simulink model "gm_uz_9ph_pmsm_model"  (R2021a)
settings: Solver=FixedStepAuto  StartTime=0.0  StopTime=.5  RelTol=1e-3
PreLoadFcn:
  | uz_pmsm_model_init_parameter
undefined symbols (not defined in the file or in its folder): friction_coefficient, inertia, k_i_d, k_p_d, k_p_q, L_d, L_o1, L_o2, L_q, L_x1, L_x2, L_y1, L_y2, L_zero, polepair, psi_pm, R_1, static_friction_torque
libraries: hdlmdlgenlib x220, hdlsllib x18, pid_lib x2, simulink x2
(part 2 of 3)

== system gm_uz_9ph_pmsm_model/uz_pmsm_model_9ph/Data Type Conversion11 ==
  In1 : Inport
  Data Type Conversion11 : DataTypeConversion  OutDataTypeStr=single  RndMeth=Nearest  SampleTime=1e-06
  Out1 : Outport
  wires:
  In1/1 -> Data Type Conversion11/1
  Data Type Conversion11/1 -> Out1/1

== system gm_uz_9ph_pmsm_model/uz_pmsm_model_9ph/Data Type Conversion111 ==
  In1 : Inport
  Data Type Conversion111 : DataTypeConversion  OutDataTypeStr=double  RndMeth=Nearest  SampleTime=1e-06
  Out1 : Outport
  wires:
  In1/1 -> Data Type Conversion111/1
  Data Type Conversion111/1 -> Out1/1

== system gm_uz_9ph_pmsm_model/uz_pmsm_model_9ph/Data Type Conversion12 ==
  In1 : Inport
  Data Type Conversion12 : DataTypeConversion  OutDataTypeStr=double  RndMeth=Nearest  SampleTime=1e-06
  Out1 : Outport
  wires:
  In1/1 -> Data Type Conversion12/1
  Data Type Conversion12/1 -> Out1/1

== system gm_uz_9ph_pmsm_model/uz_pmsm_model_9ph/Data Type Conversion121 ==
  In1 : Inport
  Data Type Conversion121 : DataTypeConversion  OutDataTypeStr=double  RndMeth=Nearest  SampleTime=1e-06
  Out1 : Outport
  wires:
  In1/1 -> Data Type Conversion121/1
  Data Type Conversion121/1 -> Out1/1

== system gm_uz_9ph_pmsm_model/uz_pmsm_model_9ph/Data Type Conversion15 ==
  In1 : Inport
  Data Type Conversion15 : DataTypeConversion  OutDataTypeStr=single  RndMeth=Nearest  SampleTime=1e-06
  Out1 : Outport
  wires:
  In1/1 -> Data Type Conversion15/1
  Data Type Conversion15/1 -> Out1/1

== system gm_uz_9ph_pmsm_model/uz_pmsm_model_9ph/Data Type Conversion16 ==
  In1 : Inport
  Data Type Conversion16 : DataTypeConversion  OutDataTypeStr=single  RndMeth=Nearest  SampleTime=1e-06
  Out1 : Outport
  wires:
  In1/1 -> Data Type Conversion16/1
  Data Type Conversion16/1 -> Out1/1

== system gm_uz_9ph_pmsm_model/uz_pmsm_model_9ph/Data Type Conversion17 ==
  In1 : Inport
  Data Type Conversion17 : DataTypeConversion  OutDataTypeStr=single  RndMeth=Nearest  SampleTime=1e-06
  Out1 : Outport
  wires:
  In1/1 -> Data Type Conversion17/1
  Data Type Conversion17/1 -> Out1/1

== system gm_uz_9ph_pmsm_model/uz_pmsm_model_9ph/Data Type Conversion18 ==
  In1 : Inport
  Data Type Conversion18 : DataTypeConversion  OutDataTypeStr=single  RndMeth=Nearest  SampleTime=1e-06
  Out1 : Outport
  wires:
  In1/1 -> Data Type Conversion18/1
  Data Type Conversion18/1 -> Out1/1

== system gm_uz_9ph_pmsm_model/uz_pmsm_model_9ph/Data Type Conversion19 ==
  In1 : Inport
  Data Type Conversion19 : DataTypeConversion  OutDataTypeStr=double  RndMeth=Nearest  SampleTime=1e-06
  Out1 : Outport
  wires:
  In1/1 -> Data Type Conversion19/1
  Data Type Conversion19/1 -> Out1/1

== system gm_uz_9ph_pmsm_model/uz_pmsm_model_9ph/Data Type Conversion2 ==
  In1 : Inport
  Data Type Conversion2 : DataTypeConversion  OutDataTypeStr=double  RndMeth=Nearest  SampleTime=1e-06
  Out1 : Outport
  wires:
  In1/1 -> Data Type Conversion2/1
  Data Type Conversion2/1 -> Out1/1

== system gm_uz_9ph_pmsm_model/uz_pmsm_model_9ph/Data Type Conversion21 ==
  In1 : Inport
  Data Type Conversion21 : DataTypeConversion  OutDataTypeStr=double  RndMeth=Nearest  SampleTime=1e-06
  Out1 : Outport
  wires:
  In1/1 -> Data Type Conversion21/1
  Data Type Conversion21/1 -> Out1/1

== system gm_uz_9ph_pmsm_model/uz_pmsm_model_9ph/Data Type Conversion26 ==
  In1 : Inport
  Data Type Conversion26 : DataTypeConversion  OutDataTypeStr=single  RndMeth=Nearest  SampleTime=1e-06
  Out1 : Outport
  wires:
  In1/1 -> Data Type Conversion26/1
  Data Type Conversion26/1 -> Out1/1

== system gm_uz_9ph_pmsm_model/uz_pmsm_model_9ph/Data Type Conversion3 ==
  In1 : Inport
  Data Type Conversion3 : DataTypeConversion  OutDataTypeStr=double  RndMeth=Nearest  SampleTime=1e-06
  Out1 : Outport
  wires:
  In1/1 -> Data Type Conversion3/1
  Data Type Conversion3/1 -> Out1/1

== system gm_uz_9ph_pmsm_model/uz_pmsm_model_9ph/Data Type Conversion30 ==
  In1 : Inport
  Data Type Conversion30 : DataTypeConversion  OutDataTypeStr=single  RndMeth=Nearest  SampleTime=1e-06
  Out1 : Outport
  wires:
  In1/1 -> Data Type Conversion30/1
  Data Type Conversion30/1 -> Out1/1

== system gm_uz_9ph_pmsm_model/uz_pmsm_model_9ph/Data Type Conversion31 ==
  In1 : Inport
  Data Type Conversion31 : DataTypeConversion  OutDataTypeStr=fixdt(1, 25, 12)  RndMeth=Nearest  SampleTime=1e-06
  Out1 : Outport
  wires:
  In1/1 -> Data Type Conversion31/1
  Data Type Conversion31/1 -> Out1/1

== system gm_uz_9ph_pmsm_model/uz_pmsm_model_9ph/Data Type Conversion32 ==
  In1 : Inport
  Data Type Conversion32 : DataTypeConversion  OutDataTypeStr=double  RndMeth=Nearest  SampleTime=1e-06
  Out1 : Outport
  wires:
  In1/1 -> Data Type Conversion32/1
  Data Type Conversion32/1 -> Out1/1

== system gm_uz_9ph_pmsm_model/uz_pmsm_model_9ph/Data Type Conversion4 ==
  In1 : Inport
  Data Type Conversion4 : DataTypeConversion  OutDataTypeStr=double  RndMeth=Nearest  SampleTime=1e-06
  Out1 : Outport
  wires:
  In1/1 -> Data Type Conversion4/1
  Data Type Conversion4/1 -> Out1/1

== system gm_uz_9ph_pmsm_model/uz_pmsm_model_9ph/Data Type Conversion41 ==
  In1 : Inport
  Data Type Conversion41 : DataTypeConversion  OutDataTypeStr=double  RndMeth=Nearest  SampleTime=1e-06
  Out1 : Outport
  wires:
  In1/1 -> Data Type Conversion41/1
  Data Type Conversion41/1 -> Out1/1

== system gm_uz_9ph_pmsm_model/uz_pmsm_model_9ph/Data Type Conversion5 ==
  In1 : Inport
  Data Type Conversion5 : DataTypeConversion  OutDataTypeStr=double  RndMeth=Nearest  SampleTime=1e-06
  Out1 : Outport
  wires:
  In1/1 -> Data Type Conversion5/1
  Data Type Conversion5/1 -> Out1/1

== system gm_uz_9ph_pmsm_model/uz_pmsm_model_9ph/Data Type Conversion51 ==
  In1 : Inport
  Data Type Conversion51 : DataTypeConversion  OutDataTypeStr=double  RndMeth=Nearest  SampleTime=1e-06
  Out1 : Outport
  wires:
  In1/1 -> Data Type Conversion51/1
  Data Type Conversion51/1 -> Out1/1

== system gm_uz_9ph_pmsm_model/uz_pmsm_model_9ph/Data Type Conversion6 ==
  In1 : Inport
  Data Type Conversion6 : DataTypeConversion  OutDataTypeStr=single  RndMeth=Nearest  SampleTime=1e-06
  Out1 : Outport
  wires:
  In1/1 -> Data Type Conversion6/1
  Data Type Conversion6/1 -> Out1/1

== system gm_uz_9ph_pmsm_model/uz_pmsm_model_9ph/Data Type Conversion61 ==
  In1 : Inport
  Data Type Conversion61 : DataTypeConversion  OutDataTypeStr=double  RndMeth=Nearest  SampleTime=1e-06
  Out1 : Outport
  wires:
  In1/1 -> Data Type Conversion61/1
  Data Type Conversion61/1 -> Out1/1

== system gm_uz_9ph_pmsm_model/uz_pmsm_model_9ph/Data Type Conversion71 ==
  In1 : Inport
  Data Type Conversion71 : DataTypeConversion  OutDataTypeStr=double  RndMeth=Nearest  SampleTime=1e-06
  Out1 : Outport
  wires:
  In1/1 -> Data Type Conversion71/1
  Data Type Conversion71/1 -> Out1/1

== system gm_uz_9ph_pmsm_model/uz_pmsm_model_9ph/Data Type Conversion8 ==
  In1 : Inport
  Data Type Conversion8 : DataTypeConversion  OutDataTypeStr=double  RndMeth=Nearest  SampleTime=1e-06
  Out1 : Outport
  wires:
  In1/1 -> Data Type Conversion8/1
  Data Type Conversion8/1 -> Out1/1

== system gm_uz_9ph_pmsm_model/uz_pmsm_model_9ph/Data Type Conversion9 ==
  In1 : Inport
  Data Type Conversion9 : DataTypeConversion  OutDataTypeStr=double  RndMeth=Nearest  SampleTime=1e-06
  Out1 : Outport
  wires:
  In1/1 -> Data Type Conversion9/1
  Data Type Conversion9/1 -> Out1/1

== system gm_uz_9ph_pmsm_model/uz_pmsm_model_9ph/Data Type Conversion91 ==
  In1 : Inport
  Data Type Conversion91 : DataTypeConversion  OutDataTypeStr=double  RndMeth=Nearest  SampleTime=1e-06
  Out1 : Outport
  wires:
  In1/1 -> Data Type Conversion91/1
  Data Type Conversion91/1 -> Out1/1

== system gm_uz_9ph_pmsm_model/uz_pmsm_model_9ph/Divide ==
  In1 : Inport
  In2 : Inport  Port=2
  Divide : Product  Inputs=**  OutDataTypeStr=double  SampleTime=1e-06
  Out1 : Outport
  wires:
  In1/1 -> Divide/1
  In2/1 -> Divide/2
  Divide/1 -> Out1/1

== system gm_uz_9ph_pmsm_model/uz_pmsm_model_9ph/Divide1 ==
  In1 : Inport
  In2 : Inport  Port=2
  Divide1 : Product  Inputs=**  OutDataTypeStr=double  SampleTime=1e-06
  Out1 : Outport
  wires:
  In1/1 -> Divide1/1
  In2/1 -> Divide1/2
  Divide1/1 -> Out1/1

== system gm_uz_9ph_pmsm_model/uz_pmsm_model_9ph/Divide10 ==
  In1 : Inport
  In2 : Inport  Port=2
  Divide10 : Product  Inputs=**  OutDataTypeStr=double  SampleTime=1e-06
  Out1 : Outport
  wires:
  In1/1 -> Divide10/1
  In2/1 -> Divide10/2
  Divide10/1 -> Out1/1

== system gm_uz_9ph_pmsm_model/uz_pmsm_model_9ph/Divide11 ==
  In1 : Inport
  In2 : Inport  Port=2
  Divide11 : Product  Inputs=*/  OutDataTypeStr=double  SampleTime=1e-06
  Out1 : Outport
  wires:
  In1/1 -> Divide11/1
  In2/1 -> Divide11/2
  Divide11/1 -> Out1/1

== system gm_uz_9ph_pmsm_model/uz_pmsm_model_9ph/Divide111 ==
  In1 : Inport
  In2 : Inport  Port=2
  Divide111 : Product  Inputs=*/  OutDataTypeStr=double  SampleTime=1e-06
  Out1 : Outport
  wires:
  In1/1 -> Divide111/1
  In2/1 -> Divide111/2
  Divide111/1 -> Out1/1

== system gm_uz_9ph_pmsm_model/uz_pmsm_model_9ph/Divide12 ==
  In1 : Inport
  In2 : Inport  Port=2
  Divide12 : Product  Inputs=**  OutDataTypeStr=double  SampleTime=1e-06
  Out1 : Outport
  wires:
  In1/1 -> Divide12/1
  In2/1 -> Divide12/2
  Divide12/1 -> Out1/1

== system gm_uz_9ph_pmsm_model/uz_pmsm_model_9ph/Divide13 ==
  In1 : Inport
  In2 : Inport  Port=2
  Divide13 : Product  Inputs=*/  OutDataTypeStr=double  SampleTime=1e-06
  Out1 : Outport
  wires:
  In1/1 -> Divide13/1
  In2/1 -> Divide13/2
  Divide13/1 -> Out1/1

== system gm_uz_9ph_pmsm_model/uz_pmsm_model_9ph/Divide2 ==
  In1 : Inport
  In2 : Inport  Port=2
  Divide2 : Product  Inputs=**  OutDataTypeStr=double  SampleTime=1e-06
  Out1 : Outport
  wires:
  In1/1 -> Divide2/1
  In2/1 -> Divide2/2
  Divide2/1 -> Out1/1

== system gm_uz_9ph_pmsm_model/uz_pmsm_model_9ph/Divide3 ==
  In1 : Inport
  In2 : Inport  Port=2
  Divide3 : Product  Inputs=*/  OutDataTypeStr=double  SampleTime=1e-06
  Out1 : Outport
  wires:
  In1/1 -> Divide3/1
  In2/1 -> Divide3/2
  Divide3/1 -> Out1/1

== system gm_uz_9ph_pmsm_model/uz_pmsm_model_9ph/Divide4 ==
  In1 : Inport
  In2 : Inport  Port=2
  Divide4 : Product  Inputs=**  OutDataTypeStr=double  SampleTime=1e-06
  Out1 : Outport
  wires:
  In1/1 -> Divide4/1
  In2/1 -> Divide4/2
  Divide4/1 -> Out1/1

== system gm_uz_9ph_pmsm_model/uz_pmsm_model_9ph/Divide5 ==
  In1 : Inport
  In2 : Inport  Port=2
  Divide5 : Product  Inputs=*/  OutDataTypeStr=double  SampleTime=1e-06
  Out1 : Outport
  wires:
  In1/1 -> Divide5/1
  In2/1 -> Divide5/2
  Divide5/1 -> Out1/1

== system gm_uz_9ph_pmsm_model/uz_pmsm_model_9ph/Divide6 ==
  In1 : Inport
  In2 : Inport  Port=2
  Divide6 : Product  Inputs=**  OutDataTypeStr=double  SampleTime=1e-06
  Out1 : Outport
  wires:
  In1/1 -> Divide6/1
  In2/1 -> Divide6/2
  Divide6/1 -> Out1/1

== system gm_uz_9ph_pmsm_model/uz_pmsm_model_9ph/Divide7 ==
  In1 : Inport
  In2 : Inport  Port=2
  Divide7 : Product  Inputs=*/  OutDataTypeStr=double  SampleTime=1e-06
  Out1 : Outport
  wires:
  In1/1 -> Divide7/1
  In2/1 -> Divide7/2
  Divide7/1 -> Out1/1

== system gm_uz_9ph_pmsm_model/uz_pmsm_model_9ph/Divide8 ==
  In1 : Inport
  In2 : Inport  Port=2
  Divide8 : Product  Inputs=**  OutDataTypeStr=double  SampleTime=1e-06
  Out1 : Outport
  wires:
  In1/1 -> Divide8/1
  In2/1 -> Divide8/2
  Divide8/1 -> Out1/1

== system gm_uz_9ph_pmsm_model/uz_pmsm_model_9ph/Divide9 ==
  In1 : Inport
  In2 : Inport  Port=2
  Divide9 : Product  Inputs=*/  OutDataTypeStr=double  SampleTime=1e-06
  Out1 : Outport
  wires:
  In1/1 -> Divide9/1
  In2/1 -> Divide9/2
  Divide9/1 -> Out1/1

== system gm_uz_9ph_pmsm_model/uz_pmsm_model_9ph/Factor ==
  In1 : Inport
  In2 : Inport  Port=2
  Factor : Product  Inputs=**  OutDataTypeStr=double  SampleTime=1e-06
  Out1 : Outport
  wires:
  In1/1 -> Factor/1
  In2/1 -> Factor/2
  Factor/1 -> Out1/1

== system gm_uz_9ph_pmsm_model/uz_pmsm_model_9ph/Gain ==
  In1 : Inport
  In2 : Inport  Port=2
  Gain : Product  Inputs=**  OutDataTypeStr=double  SampleTime=1e-06
  Out1 : Outport
  wires:
  In1/1 -> Gain/1
  In2/1 -> Gain/2
  Gain/1 -> Out1/1

== system gm_uz_9ph_pmsm_model/uz_pmsm_model_9ph/Gain1 ==
  In1 : Inport
  In2 : Inport  Port=2
  Gain1 : Product  Inputs=**  OutDataTypeStr=double  SampleTime=1e-06
  Out1 : Outport
  wires:
  In1/1 -> Gain1/1
  In2/1 -> Gain1/2
  Gain1/1 -> Out1/1

== system gm_uz_9ph_pmsm_model/uz_pmsm_model_9ph/Gain10 ==
  In1 : Inport
  In2 : Inport  Port=2
  Gain10 : Product  Inputs=**  OutDataTypeStr=double  SampleTime=1e-06
  Out1 : Outport
  wires:
  In1/1 -> Gain10/1
  In2/1 -> Gain10/2
  Gain10/1 -> Out1/1

== system gm_uz_9ph_pmsm_model/uz_pmsm_model_9ph/Gain2 ==
  In1 : Inport
  In2 : Inport  Port=2
  Gain2 : Product  Inputs=**  OutDataTypeStr=double  SampleTime=1e-06
  Out1 : Outport
  wires:
  In1/1 -> Gain2/1
  In2/1 -> Gain2/2
  Gain2/1 -> Out1/1

== system gm_uz_9ph_pmsm_model/uz_pmsm_model_9ph/Gain3 ==
  In1 : Inport
  In2 : Inport  Port=2
  Gain3 : Product  Inputs=**  OutDataTypeStr=double  SampleTime=1e-06
  Out1 : Outport
  wires:
  In1/1 -> Gain3/1
  In2/1 -> Gain3/2
  Gain3/1 -> Out1/1

== system gm_uz_9ph_pmsm_model/uz_pmsm_model_9ph/Gain4 ==
  In1 : Inport
  In2 : Inport  Port=2
  Gain4 : Product  Inputs=**  OutDataTypeStr=double  SampleTime=1e-06
  Out1 : Outport
  wires:
  In1/1 -> Gain4/1
  In2/1 -> Gain4/2
  Gain4/1 -> Out1/1

== system gm_uz_9ph_pmsm_model/uz_pmsm_model_9ph/Gain5 ==
  In1 : Inport
  In2 : Inport  Port=2
  Gain5 : Product  Inputs=**  OutDataTypeStr=double  SampleTime=1e-06
  Out1 : Outport
  wires:
  In1/1 -> Gain5/1
  In2/1 -> Gain5/2
  Gain5/1 -> Out1/1

== system gm_uz_9ph_pmsm_model/uz_pmsm_model_9ph/Gain6 ==
  In1 : Inport
  In2 : Inport  Port=2
  Gain6 : Product  Inputs=**  OutDataTypeStr=double  SampleTime=1e-06
  Out1 : Outport
  wires:
  In1/1 -> Gain6/1
  In2/1 -> Gain6/2
  Gain6/1 -> Out1/1

== system gm_uz_9ph_pmsm_model/uz_pmsm_model_9ph/Gain7 ==
  In1 : Inport
  In2 : Inport  Port=2
  Gain7 : Product  Inputs=**  OutDataTypeStr=double  SampleTime=1e-06
  Out1 : Outport
  wires:
  In1/1 -> Gain7/1
  In2/1 -> Gain7/2
  Gain7/1 -> Out1/1

== system gm_uz_9ph_pmsm_model/uz_pmsm_model_9ph/Gain8 ==
  In1 : Inport
  In2 : Inport  Port=2
  Gain8 : Product  Inputs=**  OutDataTypeStr=double  SampleTime=1e-06
  Out1 : Outport
  wires:
  In1/1 -> Gain8/1
  In2/1 -> Gain8/2
  Gain8/1 -> Out1/1

== system gm_uz_9ph_pmsm_model/uz_pmsm_model_9ph/Gain9 ==
  In1 : Inport
  In2 : Inport  Port=2
  Gain9 : Product  Inputs=**  OutDataTypeStr=double  SampleTime=1e-06
  Out1 : Outport
  wires:
  In1/1 -> Gain9/1
  In2/1 -> Gain9/2
  Gain9/1 -> Out1/1

== system gm_uz_9ph_pmsm_model/uz_pmsm_model_9ph/Product ==
  In1 : Inport
  In2 : Inport  Port=2
  Product : Product  Inputs=**  OutDataTypeStr=double  SampleTime=1e-06
  Out1 : Outport
  wires:
  In1/1 -> Product/1
  In2/1 -> Product/2
  Product/1 -> Out1/1

== system gm_uz_9ph_pmsm_model/uz_pmsm_model_9ph/Product1 ==
  In1 : Inport
  In2 : Inport  Port=2
  Product1 : Product  Inputs=**  OutDataTypeStr=double  SampleTime=1e-06
  Out1 : Outport
  wires:
  In1/1 -> Product1/1
  In2/1 -> Product1/2
  Product1/1 -> Out1/1

== system gm_uz_9ph_pmsm_model/uz_pmsm_model_9ph/Product10 ==
  In1 : Inport
  In2 : Inport  Port=2
  Product10 : Product  Inputs=**  OutDataTypeStr=double  SampleTime=1e-06
  Out1 : Outport
  wires:
  In1/1 -> Product10/1
  In2/1 -> Product10/2
  Product10/1 -> Out1/1

== system gm_uz_9ph_pmsm_model/uz_pmsm_model_9ph/Product11 ==
  In1 : Inport
  In2 : Inport  Port=2
  Product11 : Product  Inputs=**  OutDataTypeStr=double  SampleTime=1e-06
  Out1 : Outport
  wires:
  In1/1 -> Product11/1
  In2/1 -> Product11/2
  Product11/1 -> Out1/1

== system gm_uz_9ph_pmsm_model/uz_pmsm_model_9ph/Product12 ==
  In1 : Inport
  In2 : Inport  Port=2
  Product12 : Product  Inputs=**  OutDataTypeStr=double  SampleTime=1e-06
  Out1 : Outport
  wires:
  In1/1 -> Product12/1
  In2/1 -> Product12/2
  Product12/1 -> Out1/1

== system gm_uz_9ph_pmsm_model/uz_pmsm_model_9ph/Product2 ==
  In1 : Inport
  In2 : Inport  Port=2
  Product2 : Product  Inputs=**  OutDataTypeStr=double  SampleTime=1e-06
  Out1 : Outport
  wires:
  In1/1 -> Product2/1
  In2/1 -> Product2/2
  Product2/1 -> Out1/1

== system gm_uz_9ph_pmsm_model/uz_pmsm_model_9ph/Product3 ==
  In1 : Inport
  In2 : Inport  Port=2
  Product3 : Product  Inputs=**  OutDataTypeStr=double  SampleTime=1e-06
  Out1 : Outport
  wires:
  In1/1 -> Product3/1
  In2/1 -> Product3/2
  Product3/1 -> Out1/1

== system gm_uz_9ph_pmsm_model/uz_pmsm_model_9ph/Product4 ==
  In1 : Inport
  In2 : Inport  Port=2
  Product4 : Product  Inputs=**  OutDataTypeStr=double  SampleTime=1e-06
  Out1 : Outport
  wires:
  In1/1 -> Product4/1
  In2/1 -> Product4/2
  Product4/1 -> Out1/1

== system gm_uz_9ph_pmsm_model/uz_pmsm_model_9ph/Product5 ==
  In1 : Inport
  In2 : Inport  Port=2
  Product5 : Product  Inputs=**  OutDataTypeStr=double  SampleTime=1e-06
  Out1 : Outport
  wires:
  In1/1 -> Product5/1
  In2/1 -> Product5/2
  Product5/1 -> Out1/1

== system gm_uz_9ph_pmsm_model/uz_pmsm_model_9ph/Product6 ==
  In1 : Inport
  In2 : Inport  Port=2
  Product6 : Product  Inputs=**  OutDataTypeStr=double  SampleTime=1e-06
  Out1 : Outport
  wires:
  In1/1 -> Product6/1
  In2/1 -> Product6/2
  Product6/1 -> Out1/1

== system gm_uz_9ph_pmsm_model/uz_pmsm_model_9ph/Product7 ==
  In1 : Inport
  In2 : Inport  Port=2
  Product7 : Product  Inputs=**  OutDataTypeStr=double  SampleTime=1e-06
  Out1 : Outport
  wires:
  In1/1 -> Product7/1
  In2/1 -> Product7/2
  Product7/1 -> Out1/1

== system gm_uz_9ph_pmsm_model/uz_pmsm_model_9ph/Product8 ==
  In1 : Inport
  In2 : Inport  Port=2
  Product8 : Product  Inputs=**  OutDataTypeStr=double  SampleTime=1e-06
  Out1 : Outport
  wires:
  In1/1 -> Product8/1
  In2/1 -> Product8/2
  Product8/1 -> Out1/1

== system gm_uz_9ph_pmsm_model/uz_pmsm_model_9ph/Product9 ==
  In1 : Inport
  In2 : Inport  Port=2
  Product9 : Product  Inputs=**  OutDataTypeStr=double  SampleTime=1e-06
  Out1 : Outport
  wires:
  In1/1 -> Product9/1
  In2/1 -> Product9/2
  Product9/1 -> Out1/1

== system gm_uz_9ph_pmsm_model/uz_pmsm_model_9ph/Sign1 ==
  In1 : Inport
  Sign1 : Signum  SampleTime=1e-06
  Out1 : Outport
  wires:
  In1/1 -> Sign1/1
  Sign1/1 -> Out1/1

== system gm_uz_9ph_pmsm_model/uz_pmsm_model_9ph/Sum ==
  In1 : Inport
  In2 : Inport  Port=2
  Sum : Sum  Inputs=+-  OutDataTypeStr=double  SampleTime=1e-06
  Out1 : Outport
  wires:
  In1/1 -> Sum/1
  In2/1 -> Sum/2
  Sum/1 -> Out1/1

== system gm_uz_9ph_pmsm_model/uz_pmsm_model_9ph/Sum1 ==
  In1 : Inport
  In2 : Inport  Port=2
  Sum1 : Sum  Inputs=+-  OutDataTypeStr=double  SampleTime=1e-06
  Out1 : Outport
  wires:
  In1/1 -> Sum1/1
  In2/1 -> Sum1/2
  Sum1/1 -> Out1/1

== system gm_uz_9ph_pmsm_model/uz_pmsm_model_9ph/Sum1_stage2 ==
  In1 : Inport
  In2 : Inport  Port=2
  Sum1_stage2 : Sum  Inputs=+-  OutDataTypeStr=double  SampleTime=1e-06
  Out1 : Outport
  wires:
  In1/1 -> Sum1_stage2/1
  In2/1 -> Sum1_stage2/2
  Sum1_stage2/1 -> Out1/1

== system gm_uz_9ph_pmsm_model/uz_pmsm_model_9ph/Sum1_stage3 ==
  In1 : Inport
  In2 : Inport  Port=2
  Sum1_stage3 : Sum  Inputs=+-  OutDataTypeStr=double  SampleTime=1e-06
  Out1 : Outport
  wires:
  In1/1 -> Sum1_stage3/1
  In2/1 -> Sum1_stage3/2
  Sum1_stage3/1 -> Out1/1

== system gm_uz_9ph_pmsm_model/uz_pmsm_model_9ph/Sum2 ==
  In1 : Inport
  In2 : Inport  Port=2
  Sum2 : Sum  Inputs=+-  OutDataTypeStr=double  SampleTime=1e-06
  Out1 : Outport
  wires:
  In1/1 -> Sum2/1
  In2/1 -> Sum2/2
  Sum2/1 -> Out1/1

== system gm_uz_9ph_pmsm_model/uz_pmsm_model_9ph/Sum3 ==
  In1 : Inport
  In2 : Inport  Port=2
  Sum3 : Sum  OutDataTypeStr=double  SampleTime=1e-06
  Out1 : Outport
  wires:
  In1/1 -> Sum3/1
  In2/1 -> Sum3/2
  Sum3/1 -> Out1/1

== system gm_uz_9ph_pmsm_model/uz_pmsm_model_9ph/Sum31 ==
  In1 : Inport
  In2 : Inport  Port=2
  Sum31 : Sum  OutDataTypeStr=double  SampleTime=1e-06
  Out1 : Outport
  wires:
  In1/1 -> Sum31/1
  In2/1 -> Sum31/2
  Sum31/1 -> Out1/1

== system gm_uz_9ph_pmsm_model/uz_pmsm_model_9ph/Sum310 ==
  In1 : Inport
  In2 : Inport  Port=2
  Sum310 : Sum  OutDataTypeStr=double  SampleTime=1e-06
  Out1 : Outport
  wires:
  In1/1 -> Sum310/1
  In2/1 -> Sum310/2
  Sum310/1 -> Out1/1

== system gm_uz_9ph_pmsm_model/uz_pmsm_model_9ph/Sum311 ==
  In1 : Inport
  In2 : Inport  Port=2
  Sum311 : Sum  Inputs=+-  OutDataTypeStr=double  SampleTime=1e-06
  Out1 : Outport
  wires:
  In1/1 -> Sum311/1
  In2/1 -> Sum311/2
  Sum311/1 -> Out1/1

== system gm_uz_9ph_pmsm_model/uz_pmsm_model_9ph/Sum32 ==
  In1 : Inport
  In2 : Inport  Port=2
  Sum32 : Sum  OutDataTypeStr=double  SampleTime=1e-06
  Out1 : Outport
  wires:
  In1/1 -> Sum32/1
  In2/1 -> Sum32/2
  Sum32/1 -> Out1/1

== system gm_uz_9ph_pmsm_model/uz_pmsm_model_9ph/Sum33 ==
  In1 : Inport
  In2 : Inport  Port=2
  Sum33 : Sum  OutDataTypeStr=double  SampleTime=1e-06
  Out1 : Outport
  wires:
  In1/1 -> Sum33/1
  In2/1 -> Sum33/2
  Sum33/1 -> Out1/1

== system gm_uz_9ph_pmsm_model/uz_pmsm_model_9ph/Sum34 ==
  In1 : Inport
  In2 : Inport  Port=2
  Sum34 : Sum  OutDataTypeStr=double  SampleTime=1e-06
  Out1 : Outport
  wires:
  In1/1 -> Sum34/1
  In2/1 -> Sum34/2
  Sum34/1 -> Out1/1

== system gm_uz_9ph_pmsm_model/uz_pmsm_model_9ph/Sum35 ==
  In1 : Inport
  In2 : Inport  Port=2
  Sum35 : Sum  OutDataTypeStr=double  SampleTime=1e-06
  Out1 : Outport
  wires:
  In1/1 -> Sum35/1
  In2/1 -> Sum35/2
  Sum35/1 -> Out1/1

== system gm_uz_9ph_pmsm_model/uz_pmsm_model_9ph/Sum36 ==
  In1 : Inport
  In2 : Inport  Port=2
  Sum36 : Sum  OutDataTypeStr=double  SampleTime=1e-06
  Out1 : Outport
  wires:
  In1/1 -> Sum36/1
  In2/1 -> Sum36/2
  Sum36/1 -> Out1/1

== system gm_uz_9ph_pmsm_model/uz_pmsm_model_9ph/Sum37 ==
  In1 : Inport
  In2 : Inport  Port=2
  Sum37 : Sum  OutDataTypeStr=double  SampleTime=1e-06
  Out1 : Outport
  wires:
  In1/1 -> Sum37/1
  In2/1 -> Sum37/2
  Sum37/1 -> Out1/1

== system gm_uz_9ph_pmsm_model/uz_pmsm_model_9ph/Sum38 ==
  In1 : Inport
  In2 : Inport  Port=2
  Sum38 : Sum  OutDataTypeStr=double  SampleTime=1e-06
  Out1 : Outport
  wires:
  In1/1 -> Sum38/1
  In2/1 -> Sum38/2
  Sum38/1 -> Out1/1

== system gm_uz_9ph_pmsm_model/uz_pmsm_model_9ph/Sum39 ==
  In1 : Inport
  In2 : Inport  Port=2
  Sum39 : Sum  OutDataTypeStr=double  SampleTime=1e-06
  Out1 : Outport
  wires:
  In1/1 -> Sum39/1
  In2/1 -> Sum39/2
  Sum39/1 -> Out1/1

== system gm_uz_9ph_pmsm_model/uz_pmsm_model_9ph/Sum5 ==
  In1 : Inport
  In2 : Inport  Port=2
  Sum5 : Sum  OutDataTypeStr=double  SampleTime=1e-06
  Out1 : Outport
  wires:
  In1/1 -> Sum5/1
  In2/1 -> Sum5/2
  Sum5/1 -> Out1/1

== system gm_uz_9ph_pmsm_model/uz_pmsm_model_9ph/Sum_stage2 ==
  In1 : Inport
  In2 : Inport  Port=2
  Sum_stage2 : Sum  Inputs=+-  OutDataTypeStr=double  SampleTime=1e-06
  Out1 : Outport
  wires:
  In1/1 -> Sum_stage2/1
  In2/1 -> Sum_stage2/2
  Sum_stage2/1 -> Out1/1

== system gm_uz_9ph_pmsm_model/uz_pmsm_model_9ph/Sum_stage3 ==
  In1 : Inport
  In2 : Inport  Port=2
  Sum_stage3 : Sum  OutDataTypeStr=double  SampleTime=1e-06
  Out1 : Outport
  wires:
  In1/1 -> Sum_stage3/1
  In2/1 -> Sum_stage3/2
  Sum_stage3/1 -> Out1/1

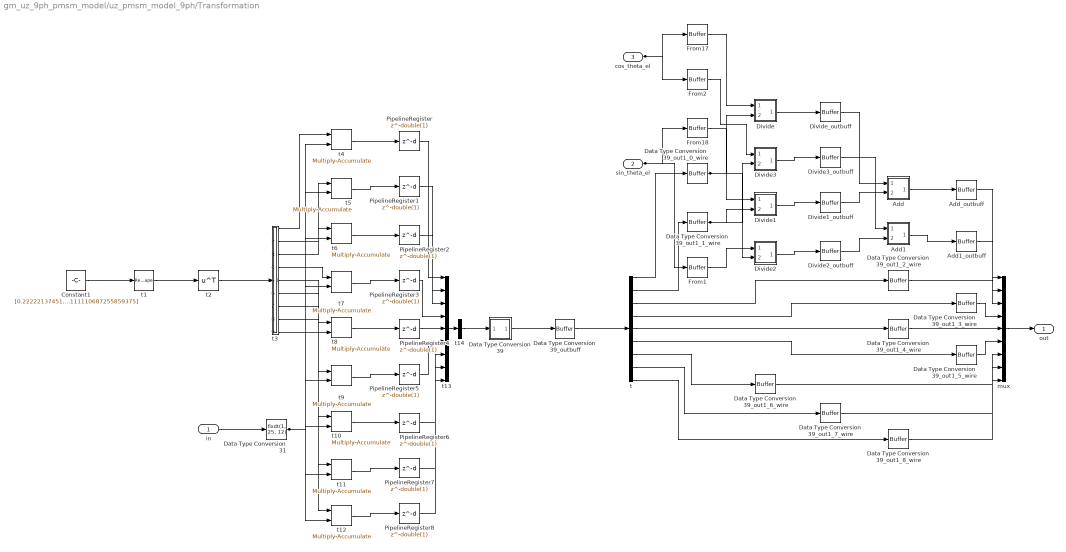
== system gm_uz_9ph_pmsm_model/uz_pmsm_model_9ph/Transformation ==
  in : Inport  OutDataTypeStr=fixdt(1, 25, 12)  PortDimensions=[9]  SampleTime=1e-06
  sin_theta_el : Inport  Port=2  OutDataTypeStr=single  SampleTime=1e-06
  cos_theta_el : Inport  Port=3  OutDataTypeStr=single  SampleTime=1e-06
  Add : Subsystem
      mask Display: disp('NFP\nadd');
  Add1 : Subsystem
      mask Display: disp('NFP\nadd');
  Add1_outbuff : hdlmdlgenlib/Buffer
      settings: SourceProductBaseCode=SL
  Add_outbuff : hdlmdlgenlib/Buffer
      settings: SourceProductBaseCode=SL
  Constant1 : Constant  Value=[0.22222137451171875;0;0.22222137451171875;0;0.22222137451171875;0;0.22222137451171875;0;0.111110687255859375;-0.111110687255859375;0.1924495697021484375;0.22222137451171875;0;-0.111110687255859375;-0.1924495697021484375;-0.111110687255859375;0.1924495697021484375;0.111110687255859375;-0.111110687255859375;-0.1924495697021484375;0.22222137451171875;0;-0.111110687255859375;0.1924495697021484375;-0.111110687255859375;-0.1924495697021484375;0.111110687255859375;0.208820343017578125;0.0760040283203125;0.111110687255859375;0.1924495697021484375;-0.0385875701904296875;0.218845367431640625;-0.1702327728271484375;0.142841339111328125;-0.111110687255859375;-0.1702327728271484375;0.142841339111328125;0.111110687255859375;0.1924495697021484375;0.208820343017578125;-0.0760040283203125;-0.0385875701904296875;-0.218845367431640625;-0.111110687255859375;-0.0385875701904296875;-0.218845367431640625;0.111110687255859375;0.1924495697021484375;-0.1702327728271484375;-0.142841339111328125;0.208820343017578125;0.0760040283203125;-0.111110687255859375;0.1702327728271484375;0.142841339111328125;-0.111110687255859375;0.1924495697021484375;-0.208820343017578125;-0.0760040283203125;0.0385875701904296875;-0.218845367431640625;0.111110687255859375;-0.208820343017578125;0.0760040283203125;-0.111110687255859375;0.1924495697021484375;0.0385875701904296875;0.218845367431640625;0.1702327728271484375;0.142841339111328125;0.111110687255859375;0.0385875701904296875;-0.218845367431640625;-0.111110687255859375;0.1924495697021484375;0.1702327728271484375;-0.142841339111328125;-0.208820343017578125;0.0760040283203125;0.111110687255859375]  OutDataTypeStr=fixdt(1, 18, 19)  SampleTime=1e-06
  Data Type Conversion31 : DataTypeConversion  OutDataTypeStr=fixdt(1, 25, 12)  RndMeth=Nearest  SampleTime=1e-06
  Data Type Conversion39 : Subsystem
      mask Display: disp('NFP\nconv');
  Data Type Conversion39_out1_0_wire : hdlmdlgenlib/Buffer
      settings: SourceProductBaseCode=SL
  Data Type Conversion39_out1_1_wire : hdlmdlgenlib/Buffer
      settings: SourceProductBaseCode=SL
  Data Type Conversion39_out1_2_wire : hdlmdlgenlib/Buffer
      settings: SourceProductBaseCode=SL
  Data Type Conversion39_out1_3_wire : hdlmdlgenlib/Buffer
      settings: SourceProductBaseCode=SL
  Data Type Conversion39_out1_4_wire : hdlmdlgenlib/Buffer
      settings: SourceProductBaseCode=SL
  Data Type Conversion39_out1_5_wire : hdlmdlgenlib/Buffer
      settings: SourceProductBaseCode=SL
  Data Type Conversion39_out1_6_wire : hdlmdlgenlib/Buffer
      settings: SourceProductBaseCode=SL
  Data Type Conversion39_out1_7_wire : hdlmdlgenlib/Buffer
      settings: SourceProductBaseCode=SL
  Data Type Conversion39_out1_8_wire : hdlmdlgenlib/Buffer
      settings: SourceProductBaseCode=SL
  Data Type Conversion39_outbuff : hdlmdlgenlib/Buffer
      settings: SourceProductBaseCode=SL
  Divide : Subsystem
      mask Display: disp('NFP\nmul');
  Divide1 : Subsystem
      mask Display: disp('NFP\nmul');
  Divide1_outbuff : hdlmdlgenlib/Buffer
      settings: SourceProductBaseCode=SL
  Divide2 : Subsystem
      mask Display: disp('NFP\nmul');
  Divide2_outbuff : hdlmdlgenlib/Buffer
      settings: SourceProductBaseCode=SL
  Divide3 : Subsystem
      mask Display: disp('NFP\nmul');
  Divide3_outbuff : hdlmdlgenlib/Buffer
      settings: SourceProductBaseCode=SL
  Divide_outbuff : hdlmdlgenlib/Buffer
      settings: SourceProductBaseCode=SL
  From{1..2,17..18} (4 alike) : hdlmdlgenlib/Buffer
      settings: SourceProductBaseCode=SL
  PipelineRegister{,1..8} (9 alike) : Delay  DelayLength=double(1)  InitialCondition=0  SampleTime=1e-06
  mux : Mux  Inputs=9
  t : Demux  Outputs=9
  t1 : Reshape  OutputDimensionality=Customize  OutputDimensions=[9,9]
  t{4..12} (9 alike) : hdlsllib/HDL Operations/Multiply-Accumulate  opMode=Vector  initValueSetting=Dialog  initValue=0  initValueSetting2=Dialog  initValue2=0  initValueSetting3=Dialog  initValue3=0  num_samples=2  RndMeth2=Floor  RndMeth3=Floor  OutDataTypeStr=fixdt(1, 43, 31)  datatype2=Inherit: Inherit via back propagation  datatype3=Inherit: Inherit via back propagation  validOut=on  endInandOut=on  startOut=on  countOut=on  dim=-1  DoSatur=off  parallel=off
      settings: SourceProductBaseCode=SL
  t13 : Mux  Inputs=9
  t14 : Concatenate  NumInputs=1  Mode=Multidimensional array  ConcatenateDimension=2
  t2 : Math  Operator=transpose  SaturateOnIntegerOverflow=on
  t3 : Subsystem
  out : Outport  SampleTime=1e-06
  wires:
  mux/1 -> out/1
  From1/1 -> Divide2/1(In1)
  From17/1 -> Divide/1(In1)
  Divide_outbuff/1 -> Add/1(In1)
  From18/1 -> Divide1/1(In1)
  Divide1_outbuff/1 -> Add/2(In2)
  From2/1 -> Divide3/1(In1)
  Divide3_outbuff/1 -> Add1/1(In1)
  t1/1 -> t2/1
  Data Type Conversion31/1 -> t12/2, t11/2, t10/2, t9/2, t8/2, t7/2, t6/2, t5/2, t4/2
  t14/1 -> Data Type Conversion39/1(In1)
  Data Type Conversion39_outbuff/1 -> t/1
  Data Type Conversion39_out1_0_wire/1 -> Divide2/2(In2), Divide/2(In2)
  Data Type Conversion39_out1_1_wire/1 -> Divide3/2(In2), Divide1/2(In2)
  Data Type Conversion39_out1_2_wire/1 -> mux/3
  Data Type Conversion39_out1_3_wire/1 -> mux/4
  Data Type Conversion39_out1_4_wire/1 -> mux/5
  Data Type Conversion39_out1_5_wire/1 -> mux/6
  Data Type Conversion39_out1_6_wire/1 -> mux/7
  Data Type Conversion39_out1_7_wire/1 -> mux/8
  Data Type Conversion39_out1_8_wire/1 -> mux/9
  Divide2_outbuff/1 -> Add1/2(In2)
  Add1_outbuff/1 -> mux/2
  Add_outbuff/1 -> mux/1
  t/1 -> Data Type Conversion39_out1_0_wire/1
  t/2 -> Data Type Conversion39_out1_1_wire/1
  t/3 -> Data Type Conversion39_out1_2_wire/1
  t/4 -> Data Type Conversion39_out1_3_wire/1
  t/5 -> Data Type Conversion39_out1_4_wire/1
  t/6 -> Data Type Conversion39_out1_5_wire/1
  t/7 -> Data Type Conversion39_out1_6_wire/1
  t/8 -> Data Type Conversion39_out1_7_wire/1
  t/9 -> Data Type Conversion39_out1_8_wire/1
  Constant1/1 -> t1/1
  t2/1 -> t3/1(in0)
  t3/1(out0) -> t4/1
  t3/2(out1) -> t5/1
  t3/3(out2) -> t6/1
  t3/4(out3) -> t7/1
  t3/5(out4) -> t8/1
  t3/6(out5) -> t9/1
  t3/7(out6) -> t10/1
  t3/8(out7) -> t11/1
  t3/9(out8) -> t12/1
  t13/1 -> t14/1
  PipelineRegister/1 -> t13/1
  PipelineRegister1/1 -> t13/2
  PipelineRegister2/1 -> t13/3
  PipelineRegister3/1 -> t13/4
  PipelineRegister4/1 -> t13/5
  PipelineRegister5/1 -> t13/6
  PipelineRegister6/1 -> t13/7
  PipelineRegister7/1 -> t13/8
  PipelineRegister8/1 -> t13/9
  Divide/1(Out1) -> Divide_outbuff/1
  Divide1/1(Out1) -> Divide1_outbuff/1
  Divide3/1(Out1) -> Divide3_outbuff/1
  Data Type Conversion39/1(Out1) -> Data Type Conversion39_outbuff/1
  Divide2/1(Out1) -> Divide2_outbuff/1
  Add1/1(Out1) -> Add1_outbuff/1
  Add/1(Out1) -> Add_outbuff/1
  in/1 -> Data Type Conversion31/1
  sin_theta_el/1 -> From1/1, From18/1
  cos_theta_el/1 -> From17/1, From2/1
  t4/1 -> PipelineRegister/1
  t5/1 -> PipelineRegister1/1
  t6/1 -> PipelineRegister2/1
  t7/1 -> PipelineRegister3/1
  t8/1 -> PipelineRegister4/1
  t9/1 -> PipelineRegister5/1
  t10/1 -> PipelineRegister6/1
  t11/1 -> PipelineRegister7/1
  t12/1 -> PipelineRegister8/1

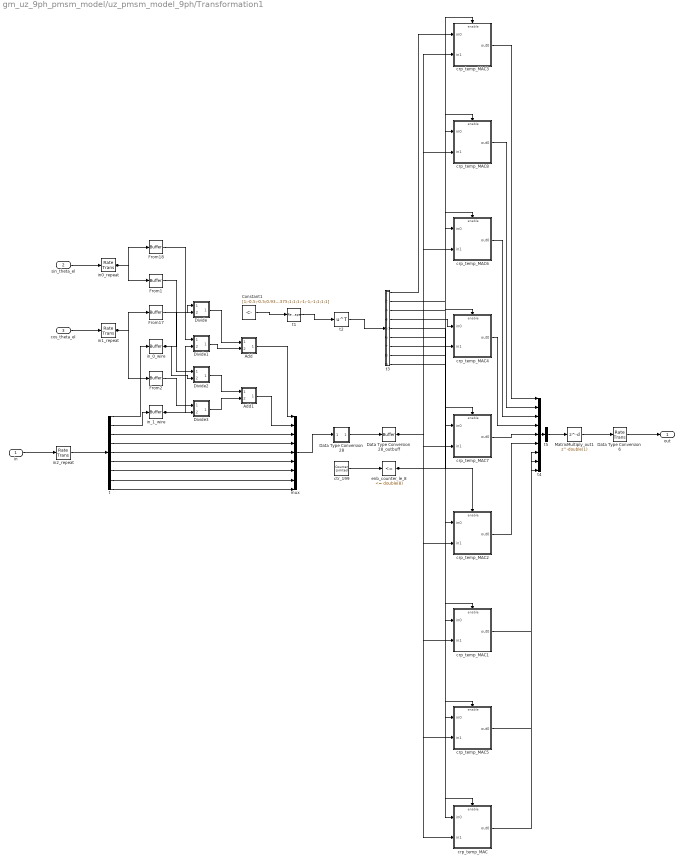
== system gm_uz_9ph_pmsm_model/uz_pmsm_model_9ph/Transformation1 ==
  in : Inport  OutDataTypeStr=single  PortDimensions=[9]  SampleTime=1e-06
  sin_theta_el : Inport  Port=2  OutDataTypeStr=single  SampleTime=1e-06
  cos_theta_el : Inport  Port=3  OutDataTypeStr=single  SampleTime=1e-06
  Add : Subsystem
      mask Display: disp('NFP\nadd');
  Add1 : Subsystem
      mask Display: disp('NFP\nadd');
  Constant1 : Constant  Value=[1;-0.5;-0.5;0.939697265625;-0.7660369873046875;-0.17364501953125;0.7660369873046875;-0.939697265625;0.17364501953125;0;0.86602783203125;-0.86602783203125;0.3420257568359375;0.642791748046875;-0.98480224609375;0.642791748046875;0.3420257568359375;-0.98480224609375;1;1;1;0.5;0.5;0.5;-0.5;-0.5;-0.5;0;0;0;0.86602783203125;0.86602783203125;0.86602783203125;0.86602783203125;0.86602783203125;0.86602783203125;1;-0.5;-0.5;-0.17364501953125;0.939697265625;-0.7660369873046875;-0.939697265625;0.17364501953125;0.7660369873046875;0;-0.86602783203125;0.86602783203125;0.98480224609375;-0.3420257568359375;-0.642791748046875;-0.3420257568359375;0.98480224609375;-0.642791748046875;1;-0.5;-0.5;-0.7660369873046875;-0.17364501953125;0.939697265625;0.17364501953125;0.7660369873046875;-0.939697265625;0;0.86602783203125;-0.86602783203125;0.642791748046875;-0.98480224609375;0.3420257568359375;-0.98480224609375;0.642791748046875;0.3420257568359375;1;1;1;-1;-1;-1;1;1;1]  OutDataTypeStr=fixdt(1, 18, 16)  SampleTime=5e-09
  Data Type Conversion28 : Subsystem
      mask Display: disp('NFP\nconv');
  Data Type Conversion28_outbuff : hdlmdlgenlib/Buffer
      settings: SourceProductBaseCode=SL
  Data Type Conversion6 : RateTransition  OutPortSampleTimeOpt=Multiple of input port sample time  OutPortSampleTimeMultiple=200
  Divide : Subsystem
      mask Display: disp('NFP\nmul');
  Divide1 : Subsystem
      mask Display: disp('NFP\nmul');
  Divide2 : Subsystem
      mask Display: disp('NFP\nmul');
  Divide3 : Subsystem
      mask Display: disp('NFP\nmul');
  From{1..2,17..18} (4 alike) : hdlmdlgenlib/Buffer
      settings: SourceProductBaseCode=SL
  MatrixMultiply_out1 : Delay  DelayLength=double(1)  InitialCondition=0  SampleTime=5e-09
  crp_temp_MAC : Subsystem
      settings: MinAlgLoopOccurrences=on
  crp_temp_MAC1 : Subsystem
      settings: MinAlgLoopOccurrences=on
  crp_temp_MAC2 : Subsystem
      settings: MinAlgLoopOccurrences=on
  crp_temp_MAC3 : Subsystem
      settings: MinAlgLoopOccurrences=on
  crp_temp_MAC4 : Subsystem
      settings: MinAlgLoopOccurrences=on
  crp_temp_MAC5 : Subsystem
      settings: MinAlgLoopOccurrences=on
  crp_temp_MAC6 : Subsystem
      settings: MinAlgLoopOccurrences=on
  crp_temp_MAC7 : Subsystem
      settings: MinAlgLoopOccurrences=on
  crp_temp_MAC8 : Subsystem
      settings: MinAlgLoopOccurrences=on
  ctr_199 : simulink/Sources/Counter Limited  uplimit=double(199)  tsamp=5e-09
  enb_counter_le_8 : simulink/Logic and Bit Operations/Compare To Constant  relop=<=  const=double(8)  OutDataTypeStr=boolean
  in0_repeat : RateTransition  Integrity=off  Deterministic=off  OutPortSampleTimeOpt=Multiple of input port sample time  OutPortSampleTimeMultiple=1/200
  in1_repeat : RateTransition  Integrity=off  Deterministic=off  OutPortSampleTimeOpt=Multiple of input port sample time  OutPortSampleTimeMultiple=1/200
  in2_repeat : RateTransition  Integrity=off  Deterministic=off  OutPortSampleTimeOpt=Multiple of input port sample time  OutPortSampleTimeMultiple=1/200
  in_0_wire : hdlmdlgenlib/Buffer
      settings: SourceProductBaseCode=SL
  in_1_wire : hdlmdlgenlib/Buffer
      settings: SourceProductBaseCode=SL
  mux : Mux  Inputs=9
  t : Demux  Outputs=9
  t1 : Reshape  OutputDimensionality=Customize  OutputDimensions=[9,9]
  t2 : Math  Operator=transpose  SaturateOnIntegerOverflow=on
  t3 : Subsystem
  t4 : Mux  Inputs=9
  t5 : Concatenate  NumInputs=1  Mode=Multidimensional array  ConcatenateDimension=2
  out : Outport  SampleTime=1e-06
  wires:
  in/1 -> in2_repeat/1
  sin_theta_el/1 -> in0_repeat/1
  cos_theta_el/1 -> in1_repeat/1
  Data Type Conversion6/1 -> out/1
  MatrixMultiply_out1/1 -> Data Type Conversion6/1
  in0_repeat/1 -> From1/1, From18/1
  in1_repeat/1 -> From17/1, From2/1
  in2_repeat/1 -> t/1
  t1/1 -> t2/1
  Data Type Conversion28_outbuff/1 -> crp_temp_MAC3/2(in1), crp_temp_MAC8/2(in1), crp_temp_MAC6/2(in1), crp_temp_MAC4/2(in1), crp_temp_MAC7/2(in1), crp_temp_MAC2/2(in1), crp_temp_MAC1/2(in1), crp_temp_MAC5/2(in1), crp_temp_MAC/2(in1)
  From1/1 -> Divide2/1(In1)
  From17/1 -> Divide/1(In1)
  From2/1 -> Divide3/1(In1)
  From18/1 -> Divide1/1(In1)
  in_0_wire/1 -> Divide2/2(In2), Divide/2(In2)
  in_1_wire/1 -> Divide1/2(In2), Divide3/2(In2)
  mux/1 -> Data Type Conversion28/1(In1)
  t5/1 -> MatrixMultiply_out1/1
  t/1 -> in_0_wire/1
  t/2 -> in_1_wire/1
  t/3 -> mux/3
  t/4 -> mux/4
  t/5 -> mux/5
  t/6 -> mux/6
  t/7 -> mux/7
  t/8 -> mux/8
  t/9 -> mux/9
  Constant1/1 -> t1/1
  t2/1 -> t3/1(in0)
  t3/1(out0) -> crp_temp_MAC3/1(in0)
  t3/2(out1) -> crp_temp_MAC8/1(in0)
  t3/3(out2) -> crp_temp_MAC6/1(in0)
  t3/4(out3) -> crp_temp_MAC4/1(in0)
  t3/5(out4) -> crp_temp_MAC7/1(in0)
  t3/6(out5) -> crp_temp_MAC2/1(in0)
  t3/7(out6) -> crp_temp_MAC1/1(in0)
  t3/8(out7) -> crp_temp_MAC5/1(in0)
  t3/9(out8) -> crp_temp_MAC/1(in0)
  crp_temp_MAC3/1(out0) -> t4/1
  crp_temp_MAC8/1(out0) -> t4/2
  crp_temp_MAC6/1(out0) -> t4/3
  crp_temp_MAC4/1(out0) -> t4/4
  crp_temp_MAC7/1(out0) -> t4/5
  crp_temp_MAC2/1(out0) -> t4/6
  crp_temp_MAC1/1(out0) -> t4/7
  crp_temp_MAC5/1(out0) -> t4/8
  crp_temp_MAC/1(out0) -> t4/9
  t4/1 -> t5/1
  Data Type Conversion28/1(Out1) -> Data Type Conversion28_outbuff/1
  Divide/1(Out1) -> Add/1(In1)
  Divide3/1(Out1) -> Add1/2(In2)
  Divide1/1(Out1) -> Add/2(In2)
  Divide2/1(Out1) -> Add1/1(In1)
  Add1/1(Out1) -> mux/2
  Add/1(Out1) -> mux/1
  enb_counter_le_8/1 -> crp_temp_MAC3/Enable, crp_temp_MAC8/Enable, crp_temp_MAC6/Enable, crp_temp_MAC4/Enable, crp_temp_MAC7/Enable, crp_temp_MAC2/Enable, crp_temp_MAC1/Enable, crp_temp_MAC5/Enable, crp_temp_MAC/Enable
  ctr_199/1 -> enb_counter_le_8/1

== system gm_uz_9ph_pmsm_model/uz_pmsm_model_9ph/Transformation/Add ==
  In1 : Inport
  In2 : Inport  Port=2
  Add : Sum  OutDataTypeStr=single  SampleTime=1e-06
  Out1 : Outport
  wires:
  In1/1 -> Add/1
  In2/1 -> Add/2
  Add/1 -> Out1/1

== system gm_uz_9ph_pmsm_model/uz_pmsm_model_9ph/Transformation/Add1 ==
  In1 : Inport
  In2 : Inport  Port=2
  Add1 : Sum  Inputs=+-  OutDataTypeStr=single  SampleTime=1e-06
  Out1 : Outport
  wires:
  In1/1 -> Add1/1
  In2/1 -> Add1/2
  Add1/1 -> Out1/1

== system gm_uz_9ph_pmsm_model/uz_pmsm_model_9ph/Transformation/Data Type Conversion39 ==
  In1 : Inport
  Data Type Conversion39 : DataTypeConversion  OutDataTypeStr=single  RndMeth=Nearest  SampleTime=1e-06
  Out1 : Outport
  wires:
  In1/1 -> Data Type Conversion39/1
  Data Type Conversion39/1 -> Out1/1

== system gm_uz_9ph_pmsm_model/uz_pmsm_model_9ph/Transformation/Divide ==
  In1 : Inport
  In2 : Inport  Port=2
  Divide : Product  Inputs=**  OutDataTypeStr=single  SampleTime=1e-06
  Out1 : Outport
  wires:
  In1/1 -> Divide/1
  In2/1 -> Divide/2
  Divide/1 -> Out1/1

== system gm_uz_9ph_pmsm_model/uz_pmsm_model_9ph/Transformation/Divide1 ==
  In1 : Inport
  In2 : Inport  Port=2
  Divide1 : Product  Inputs=**  OutDataTypeStr=single  SampleTime=1e-06
  Out1 : Outport
  wires:
  In1/1 -> Divide1/1
  In2/1 -> Divide1/2
  Divide1/1 -> Out1/1

== system gm_uz_9ph_pmsm_model/uz_pmsm_model_9ph/Transformation/Divide2 ==
  In1 : Inport
  In2 : Inport  Port=2
  Divide2 : Product  Inputs=**  OutDataTypeStr=single  SampleTime=1e-06
  Out1 : Outport
  wires:
  In1/1 -> Divide2/1
  In2/1 -> Divide2/2
  Divide2/1 -> Out1/1

== system gm_uz_9ph_pmsm_model/uz_pmsm_model_9ph/Transformation/Divide3 ==
  In1 : Inport
  In2 : Inport  Port=2
  Divide3 : Product  Inputs=**  OutDataTypeStr=single  SampleTime=1e-06
  Out1 : Outport
  wires:
  In1/1 -> Divide3/1
  In2/1 -> Divide3/2
  Divide3/1 -> Out1/1

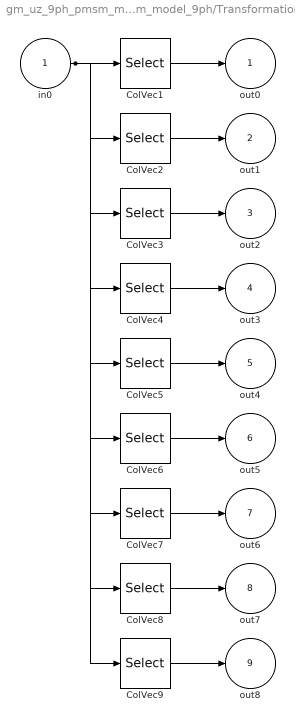
== system gm_uz_9ph_pmsm_model/uz_pmsm_model_9ph/Transformation/t3 ==
  in0 : Inport
  ColVec1 : Selector  NumberOfDimensions=2  IndexOptions=Select all,Index vector (dialog)  Indices=1,1  OutputSizes=1,1
  ColVec2 : Selector  NumberOfDimensions=2  IndexOptions=Select all,Index vector (dialog)  Indices=1,2  OutputSizes=1,1
  ColVec3 : Selector  NumberOfDimensions=2  IndexOptions=Select all,Index vector (dialog)  Indices=1,3  OutputSizes=1,1
  ColVec4 : Selector  NumberOfDimensions=2  IndexOptions=Select all,Index vector (dialog)  Indices=1,4  OutputSizes=1,1
  ColVec5 : Selector  NumberOfDimensions=2  IndexOptions=Select all,Index vector (dialog)  Indices=1,5  OutputSizes=1,1
  ColVec6 : Selector  NumberOfDimensions=2  IndexOptions=Select all,Index vector (dialog)  Indices=1,6  OutputSizes=1,1
  ColVec7 : Selector  NumberOfDimensions=2  IndexOptions=Select all,Index vector (dialog)  Indices=1,7  OutputSizes=1,1
  ColVec8 : Selector  NumberOfDimensions=2  IndexOptions=Select all,Index vector (dialog)  Indices=1,8  OutputSizes=1,1
  ColVec9 : Selector  NumberOfDimensions=2  IndexOptions=Select all,Index vector (dialog)  Indices=1,9  OutputSizes=1,1
  out0 : Outport
  out1 : Outport  Port=2
  out2 : Outport  Port=3
  out3 : Outport  Port=4
  out4 : Outport  Port=5
  out5 : Outport  Port=6
  out6 : Outport  Port=7
  out7 : Outport  Port=8
  out8 : Outport  Port=9
  wires:
  in0/1 -> ColVec1/1, ColVec2/1, ColVec3/1, ColVec4/1, ColVec5/1, ColVec6/1, ColVec7/1, ColVec8/1, ColVec9/1
  ColVec1/1 -> out0/1
  ColVec2/1 -> out1/1
  ColVec3/1 -> out2/1
  ColVec4/1 -> out3/1
  ColVec5/1 -> out4/1
  ColVec6/1 -> out5/1
  ColVec7/1 -> out6/1
  ColVec8/1 -> out7/1
  ColVec9/1 -> out8/1

== system gm_uz_9ph_pmsm_model/uz_pmsm_model_9ph/Transformation1/Add ==
  In1 : Inport
  In2 : Inport  Port=2
  Add : Sum  Inputs=+-  OutDataTypeStr=single  SampleTime=5e-09
  Out1 : Outport
  wires:
  In1/1 -> Add/1
  In2/1 -> Add/2
  Add/1 -> Out1/1

== system gm_uz_9ph_pmsm_model/uz_pmsm_model_9ph/Transformation1/Add1 ==
  In1 : Inport
  In2 : Inport  Port=2
  Add1 : Sum  OutDataTypeStr=single  SampleTime=5e-09
  Out1 : Outport
  wires:
  In1/1 -> Add1/1
  In2/1 -> Add1/2
  Add1/1 -> Out1/1

== system gm_uz_9ph_pmsm_model/uz_pmsm_model_9ph/Transformation1/Data Type Conversion28 ==
  In1 : Inport
  Data Type Conversion28 : DataTypeConversion  OutDataTypeStr=fixdt(1, 25, 12)  RndMeth=Nearest  SampleTime=5e-09
  Out1 : Outport
  wires:
  In1/1 -> Data Type Conversion28/1
  Data Type Conversion28/1 -> Out1/1

== system gm_uz_9ph_pmsm_model/uz_pmsm_model_9ph/Transformation1/Divide ==
  In1 : Inport
  In2 : Inport  Port=2
  Divide : Product  Inputs=**  OutDataTypeStr=single  SampleTime=5e-09
  Out1 : Outport
  wires:
  In1/1 -> Divide/1
  In2/1 -> Divide/2
  Divide/1 -> Out1/1

== system gm_uz_9ph_pmsm_model/uz_pmsm_model_9ph/Transformation1/Divide1 ==
  In1 : Inport
  In2 : Inport  Port=2
  Divide1 : Product  Inputs=**  OutDataTypeStr=single  SampleTime=5e-09
  Out1 : Outport
  wires:
  In1/1 -> Divide1/1
  In2/1 -> Divide1/2
  Divide1/1 -> Out1/1

== system gm_uz_9ph_pmsm_model/uz_pmsm_model_9ph/Transformation1/Divide2 ==
  In1 : Inport
  In2 : Inport  Port=2
  Divide2 : Product  Inputs=**  OutDataTypeStr=single  SampleTime=5e-09
  Out1 : Outport
  wires:
  In1/1 -> Divide2/1
  In2/1 -> Divide2/2
  Divide2/1 -> Out1/1

== system gm_uz_9ph_pmsm_model/uz_pmsm_model_9ph/Transformation1/Divide3 ==
  In1 : Inport
  In2 : Inport  Port=2
  Divide3 : Product  Inputs=**  OutDataTypeStr=single  SampleTime=5e-09
  Out1 : Outport
  wires:
  In1/1 -> Divide3/1
  In2/1 -> Divide3/2
  Divide3/1 -> Out1/1

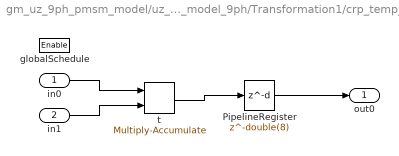
== system gm_uz_9ph_pmsm_model/uz_pmsm_model_9ph/Transformation1/crp_temp_MAC ==
  in0 : Inport  OutDataTypeStr=fixdt(1, 18, 16)  PortDimensions=[9 1]  SampleTime=5e-09
  in1 : Inport  Port=2  OutDataTypeStr=fixdt(1, 25, 12)  PortDimensions=[9]  SampleTime=5e-09
  globalSchedule : EnablePort  OutDataTypeStr=boolean
  PipelineRegister : Delay  DelayLength=double(8)  InitialCondition=0
  t : hdlsllib/HDL Operations/Multiply-Accumulate  opMode=Vector  initValueSetting=Dialog  initValue=0  initValueSetting2=Dialog  initValue2=0  initValueSetting3=Dialog  initValue3=0  num_samples=2  RndMeth2=Floor  RndMeth3=Floor  OutDataTypeStr=fixdt(1, 43, 28)  datatype2=Inherit: Inherit via back propagation  datatype3=Inherit: Inherit via back propagation  validOut=on  endInandOut=on  startOut=on  countOut=on  dim=-1  DoSatur=off  parallel=off
      settings: SourceProductBaseCode=SL
  out0 : Outport  OutDataTypeStr=fixdt(1, 43, 28)  SampleTime=5e-09  InitialOutput=0
  wires:
  PipelineRegister/1 -> out0/1
  in0/1 -> t/1
  in1/1 -> t/2
  t/1 -> PipelineRegister/1

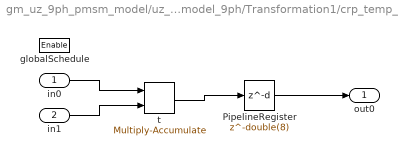
== system gm_uz_9ph_pmsm_model/uz_pmsm_model_9ph/Transformation1/crp_temp_MAC1 ==
  in0 : Inport  OutDataTypeStr=fixdt(1, 18, 16)  PortDimensions=[9 1]  SampleTime=5e-09
  in1 : Inport  Port=2  OutDataTypeStr=fixdt(1, 25, 12)  PortDimensions=[9]  SampleTime=5e-09
  globalSchedule : EnablePort  OutDataTypeStr=boolean
  PipelineRegister : Delay  DelayLength=double(8)  InitialCondition=0
  t : hdlsllib/HDL Operations/Multiply-Accumulate  opMode=Vector  initValueSetting=Dialog  initValue=0  initValueSetting2=Dialog  initValue2=0  initValueSetting3=Dialog  initValue3=0  num_samples=2  RndMeth2=Floor  RndMeth3=Floor  OutDataTypeStr=fixdt(1, 43, 28)  datatype2=Inherit: Inherit via back propagation  datatype3=Inherit: Inherit via back propagation  validOut=on  endInandOut=on  startOut=on  countOut=on  dim=-1  DoSatur=off  parallel=off
      settings: SourceProductBaseCode=SL
  out0 : Outport  OutDataTypeStr=fixdt(1, 43, 28)  SampleTime=5e-09  InitialOutput=0
  wires:
  PipelineRegister/1 -> out0/1
  in0/1 -> t/1
  in1/1 -> t/2
  t/1 -> PipelineRegister/1

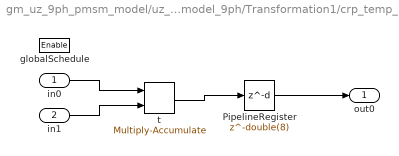
== system gm_uz_9ph_pmsm_model/uz_pmsm_model_9ph/Transformation1/crp_temp_MAC2 ==
  in0 : Inport  OutDataTypeStr=fixdt(1, 18, 16)  PortDimensions=[9 1]  SampleTime=5e-09
  in1 : Inport  Port=2  OutDataTypeStr=fixdt(1, 25, 12)  PortDimensions=[9]  SampleTime=5e-09
  globalSchedule : EnablePort  OutDataTypeStr=boolean
  PipelineRegister : Delay  DelayLength=double(8)  InitialCondition=0
  t : hdlsllib/HDL Operations/Multiply-Accumulate  opMode=Vector  initValueSetting=Dialog  initValue=0  initValueSetting2=Dialog  initValue2=0  initValueSetting3=Dialog  initValue3=0  num_samples=2  RndMeth2=Floor  RndMeth3=Floor  OutDataTypeStr=fixdt(1, 43, 28)  datatype2=Inherit: Inherit via back propagation  datatype3=Inherit: Inherit via back propagation  validOut=on  endInandOut=on  startOut=on  countOut=on  dim=-1  DoSatur=off  parallel=off
      settings: SourceProductBaseCode=SL
  out0 : Outport  OutDataTypeStr=fixdt(1, 43, 28)  SampleTime=5e-09  InitialOutput=0
  wires:
  PipelineRegister/1 -> out0/1
  in0/1 -> t/1
  in1/1 -> t/2
  t/1 -> PipelineRegister/1

== system gm_uz_9ph_pmsm_model/uz_pmsm_model_9ph/Transformation1/crp_temp_MAC3 ==
  in0 : Inport  OutDataTypeStr=fixdt(1, 18, 16)  PortDimensions=[9 1]  SampleTime=5e-09
  in1 : Inport  Port=2  OutDataTypeStr=fixdt(1, 25, 12)  PortDimensions=[9]  SampleTime=5e-09
  globalSchedule : EnablePort  OutDataTypeStr=boolean
  PipelineRegister : Delay  DelayLength=double(8)  InitialCondition=0
  t : hdlsllib/HDL Operations/Multiply-Accumulate  opMode=Vector  initValueSetting=Dialog  initValue=0  initValueSetting2=Dialog  initValue2=0  initValueSetting3=Dialog  initValue3=0  num_samples=2  RndMeth2=Floor  RndMeth3=Floor  OutDataTypeStr=fixdt(1, 43, 28)  datatype2=Inherit: Inherit via back propagation  datatype3=Inherit: Inherit via back propagation  validOut=on  endInandOut=on  startOut=on  countOut=on  dim=-1  DoSatur=off  parallel=off
      settings: SourceProductBaseCode=SL
  out0 : Outport  OutDataTypeStr=fixdt(1, 43, 28)  SampleTime=5e-09  InitialOutput=0
  wires:
  PipelineRegister/1 -> out0/1
  in0/1 -> t/1
  in1/1 -> t/2
  t/1 -> PipelineRegister/1

== system gm_uz_9ph_pmsm_model/uz_pmsm_model_9ph/Transformation1/crp_temp_MAC4 ==
  in0 : Inport  OutDataTypeStr=fixdt(1, 18, 16)  PortDimensions=[9 1]  SampleTime=5e-09
  in1 : Inport  Port=2  OutDataTypeStr=fixdt(1, 25, 12)  PortDimensions=[9]  SampleTime=5e-09
  globalSchedule : EnablePort  OutDataTypeStr=boolean
  PipelineRegister : Delay  DelayLength=double(8)  InitialCondition=0
  t : hdlsllib/HDL Operations/Multiply-Accumulate  opMode=Vector  initValueSetting=Dialog  initValue=0  initValueSetting2=Dialog  initValue2=0  initValueSetting3=Dialog  initValue3=0  num_samples=2  RndMeth2=Floor  RndMeth3=Floor  OutDataTypeStr=fixdt(1, 43, 28)  datatype2=Inherit: Inherit via back propagation  datatype3=Inherit: Inherit via back propagation  validOut=on  endInandOut=on  startOut=on  countOut=on  dim=-1  DoSatur=off  parallel=off
      settings: SourceProductBaseCode=SL
  out0 : Outport  OutDataTypeStr=fixdt(1, 43, 28)  SampleTime=5e-09  InitialOutput=0
  wires:
  PipelineRegister/1 -> out0/1
  in0/1 -> t/1
  in1/1 -> t/2
  t/1 -> PipelineRegister/1

== system gm_uz_9ph_pmsm_model/uz_pmsm_model_9ph/Transformation1/crp_temp_MAC5 ==
  in0 : Inport  OutDataTypeStr=fixdt(1, 18, 16)  PortDimensions=[9 1]  SampleTime=5e-09
  in1 : Inport  Port=2  OutDataTypeStr=fixdt(1, 25, 12)  PortDimensions=[9]  SampleTime=5e-09
  globalSchedule : EnablePort  OutDataTypeStr=boolean
  PipelineRegister : Delay  DelayLength=double(8)  InitialCondition=0
  t : hdlsllib/HDL Operations/Multiply-Accumulate  opMode=Vector  initValueSetting=Dialog  initValue=0  initValueSetting2=Dialog  initValue2=0  initValueSetting3=Dialog  initValue3=0  num_samples=2  RndMeth2=Floor  RndMeth3=Floor  OutDataTypeStr=fixdt(1, 43, 28)  datatype2=Inherit: Inherit via back propagation  datatype3=Inherit: Inherit via back propagation  validOut=on  endInandOut=on  startOut=on  countOut=on  dim=-1  DoSatur=off  parallel=off
      settings: SourceProductBaseCode=SL
  out0 : Outport  OutDataTypeStr=fixdt(1, 43, 28)  SampleTime=5e-09  InitialOutput=0
  wires:
  PipelineRegister/1 -> out0/1
  in0/1 -> t/1
  in1/1 -> t/2
  t/1 -> PipelineRegister/1
